simulink model "dataLoggerSimulink"  (R2023b)
settings: Solver=FixedStepDiscrete  StartTime=0.0  StopTime=10  FixedStep=50e-6  RelTol=1e-3
undefined symbols (not defined in the file or in its folder): A1, B1, fc, gamma, H1, H2, h3, J_dsmo, P, Te
libraries: embmathops x2
settings Model: Creator=salhajhass  LastModifiedBy=rdelpoux

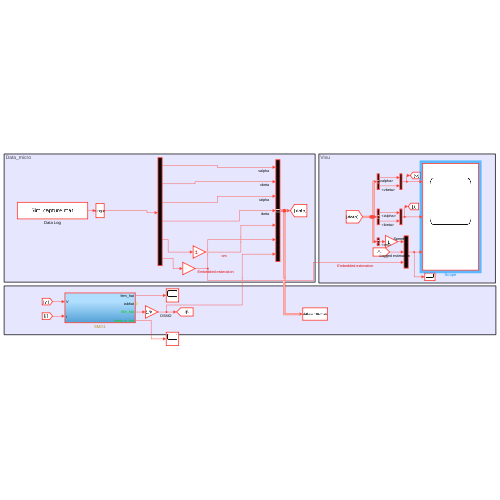
[thumbnail: Simulink's stored preview of the top-level diagram]
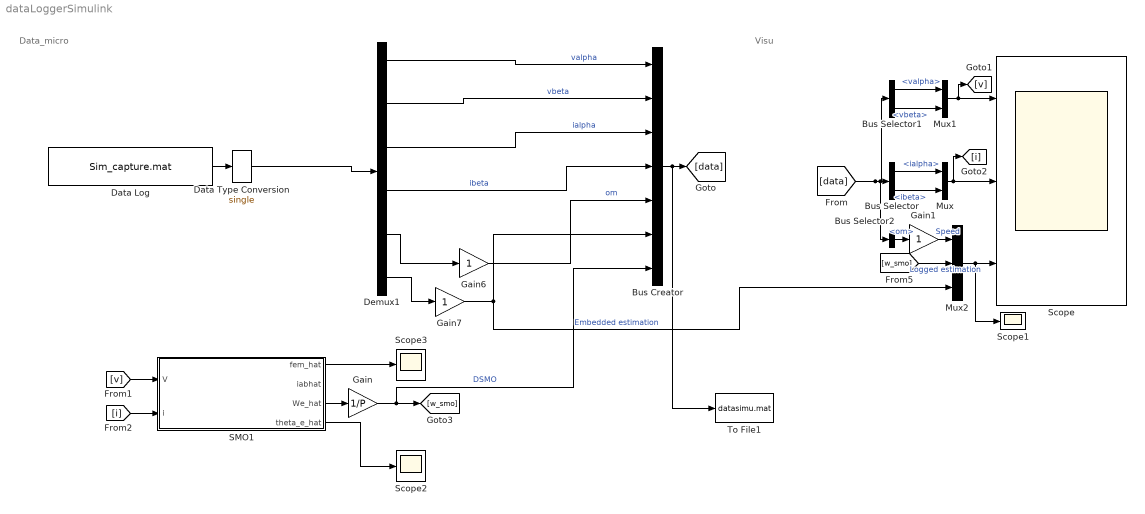
== system dataLoggerSimulink ==
  note: Visu
  note: Data_micro
  Bus Creator : BusCreator  Inputs=7
  Bus Selector : BusSelector  OutputSignals=ialpha,ibeta
  Bus Selector1 : BusSelector  OutputSignals=valpha,vbeta
  Bus Selector2 : BusSelector  OutputSignals=om
  Data Log : FromFile  FileName=Sim_capture.mat  SampleTime=50e-6
  Data Type Conversion : DataTypeConversion  OutDataTypeStr=single  SaturateOnIntegerOverflow=off  RndMeth=Floor
  Demux1 : Demux  Outputs=6
  Gain : Gain  Gain=1/P
  Gain1 : Gain
  Gain6 : Gain  OutDataTypeStr=single
  Gain7 : Gain  OutDataTypeStr=single
  Mux : Mux  Inputs=2
  Mux1 : Mux  Inputs=2
  Mux2 : Mux  Inputs=3
  SMO1 : Subsystem
  Scope : Scope  NumInputPorts=3
  Scope1 : Scope
  Scope2 : Scope
  Scope3 : Scope
  To File1 : ToFile  Filename=datasimu.mat  SaveFormat=Timeseries  SampleTime=5e-5
  wires:
  Data Log/1 -> Data Type Conversion/1
  Demux1/5 -> Gain6/1
  Bus Creator/1 -> To File1/1, [data]
  Bus Selector/1 -> Mux/1  "<ialpha>"
  Bus Selector/2 -> Mux/2  "<ibeta>"
  Mux/1 -> [i], Scope/2
  Mux1/1 -> [v], Scope/1
  Bus Selector1/2 -> Mux1/2  "<vbeta>"
  Bus Selector1/1 -> Mux1/1  "<valpha>"
  [data] -> Bus Selector1/1, Bus Selector2/1, Bus Selector/1
  Mux2/1 -> Scope1/1, Scope/3
  SMO1/3(We_hat) -> Gain/1
  Gain6/1 -> Bus Creator/5  "om"
  [v] -> SMO1/1(V)
  [i] -> SMO1/2(i)
  Gain/1 -> Bus Creator/7, [w_smo]  "DSMO"
  [w_smo] -> Mux2/2  "Logged estimation"
  Data Type Conversion/1 -> Demux1/1
  Demux1/3 -> Bus Creator/3  "ialpha"
  Demux1/4 -> Bus Creator/4  "ibeta"
  Demux1/2 -> Bus Creator/2  "vbeta"
  Demux1/1 -> Bus Creator/1  "valpha"
  Demux1/6 -> Gain7/1
  Gain7/1 -> Bus Creator/6, Mux2/3  "Embedded estimation"
  SMO1/1(fem_hat) -> Scope3/1
  Bus Selector2/1 -> Gain1/1  "<om>"
  Gain1/1 -> Mux2/1  "Speed"
  SMO1/4(theta_e_hat) -> Scope2/1

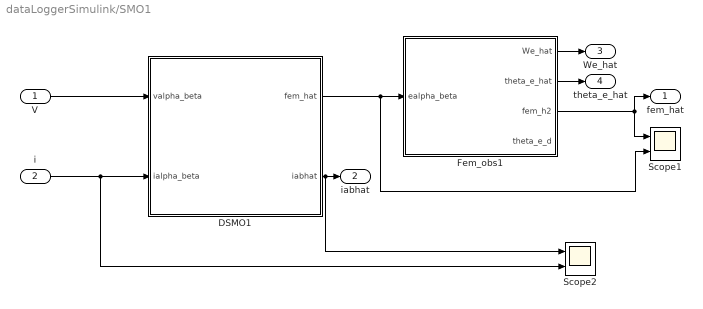
== system dataLoggerSimulink/SMO1 ==
  V : Inport
  i : Inport  Port=2
  DSMO1 : Subsystem
  Fem_obs1 : Subsystem
  Scope1 : Scope  NumInputPorts=2
  Scope2 : Scope  NumInputPorts=2
  fem_hat : Outport
  iabhat : Outport  Port=2
  We_hat : Outport  Port=3
  theta_e_hat : Outport  Port=4
  wires:
  Fem_obs1/3(fem_h2) -> fem_hat/1, Scope1/1
  Fem_obs1/2(theta_e_hat) -> theta_e_hat/1
  Fem_obs1/1(We_hat) -> We_hat/1
  i/1 -> Scope2/2, DSMO1/2(ialpha_beta)
  V/1 -> DSMO1/1(valpha_beta)
  DSMO1/2(iabhat) -> Scope2/1, iabhat/1
  DSMO1/1(fem_hat) -> Fem_obs1/1(ealpha_beta), Scope1/2

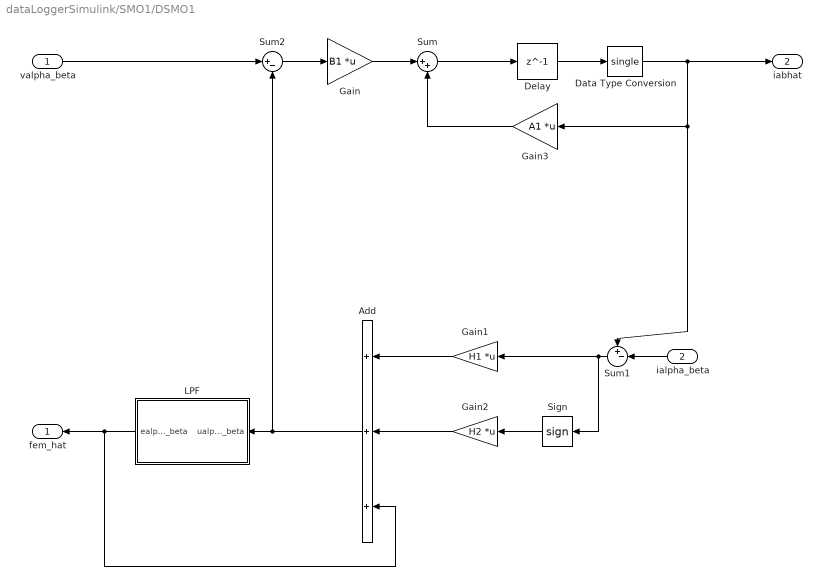
== system dataLoggerSimulink/SMO1/DSMO1 ==
  valpha_beta : Inport
  ialpha_beta : Inport  Port=2
  Add : Sum  Inputs=+++
  Data Type Conversion : DataTypeConversion  OutDataTypeStr=single  SaturateOnIntegerOverflow=off  RndMeth=Floor
  Delay : Delay  DelayLength=1  InitialCondition=0  SampleTime=Te
  Gain : Gain  Gain=B1  Multiplication=Matrix(K*u)
  Gain1 : Gain  Gain=H1  Multiplication=Matrix(K*u)
  Gain2 : Gain  Gain=H2  Multiplication=Matrix(K*u)
  Gain3 : Gain  Gain=A1  Multiplication=Matrix(K*u)
  LPF : Subsystem
  Sign : Signum
  Sum : Sum  Inputs=|++
  Sum1 : Sum  Inputs=+-|
  Sum2 : Sum  Inputs=|+-
  fem_hat : Outport
  iabhat : Outport  Port=2
  wires:
  Data Type Conversion/1 -> Gain3/1, Sum1/1, iabhat/1
  Delay/1 -> Data Type Conversion/1
  Add/1 -> Sum2/2, LPF/1(ualpha_beta)
  LPF/1(ealpha_beta) -> fem_hat/1, Add/3
  Gain2/1 -> Add/2
  Sign/1 -> Gain2/1
  Gain1/1 -> Add/1
  Sum1/1 -> Gain1/1, Sign/1
  valpha_beta/1 -> Sum2/1
  Sum2/1 -> Gain/1
  ialpha_beta/1 -> Sum1/2
  Gain3/1 -> Sum/2
  Gain/1 -> Sum/1
  Sum/1 -> Delay/1

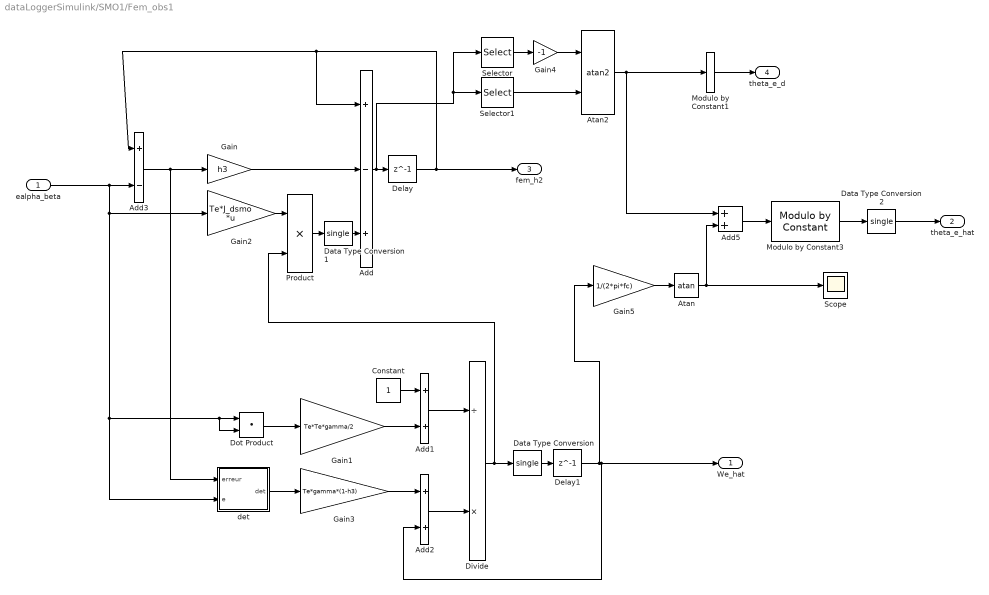
== system dataLoggerSimulink/SMO1/Fem_obs1 ==
  ealpha_beta : Inport
  Add : Sum  Inputs=+-+
  Add1 : Sum
  Add2 : Sum
  Add3 : Sum  Inputs=+-
  Add5 : Sum
  Atan : Trigonometry  Operator=atan
  Atan2 : Trigonometry  Operator=atan2  ApproximationMethod=Lookup  NumberOfDataPoints=32
  Constant : Constant
  Data Type Conversion : DataTypeConversion  OutDataTypeStr=single  SaturateOnIntegerOverflow=off  RndMeth=Floor
  Data Type Conversion1 : DataTypeConversion  OutDataTypeStr=single  SaturateOnIntegerOverflow=off  RndMeth=Floor
  Data Type Conversion2 : DataTypeConversion  OutDataTypeStr=single  SaturateOnIntegerOverflow=off  RndMeth=Floor
  Delay : Delay  DelayLength=1  SampleTime=Te
  Delay1 : Delay  DelayLength=1  SampleTime=Te
  Divide : Product  Inputs=/*
  Dot Product : DotProduct  OutDataTypeStr=Inherit: Inherit via internal rule
  Gain : Gain  Gain=h3
  Gain1 : Gain  Gain=Te*Te*gamma/2
  Gain2 : Gain  Gain=Te*J_dsmo  Multiplication=Matrix(K*u)
  Gain3 : Gain  Gain=Te*gamma*(1-h3)
  Gain4 : Gain  Gain=-1
  Gain5 : Gain  Gain=1/(2*pi*fc)
  Modulo by Constant1 : embmathops/Modulo by Constant  Denominator=2*pi  SimulateUsing=Code generation
      settings: LibrarySourceBlock=embeddedMathLib/Modulo by Constant
  Modulo by Constant3 : embmathops/Modulo by Constant  Denominator=2*pi  SimulateUsing=Code generation
      settings: LibrarySourceBlock=embeddedMathLib/Modulo by Constant
  Product : Product
  Scope : Scope
  Selector : Selector  InputPortWidth=2  IndexOptions=Index vector (dialog)  Indices=[1]  OutputSizes=1
  Selector1 : Selector  InputPortWidth=2  IndexOptions=Index vector (dialog)  Indices=2  OutputSizes=1
  det : Subsystem
  We_hat : Outport
  theta_e_hat : Outport  Port=2
  fem_h2 : Outport  Port=3
  theta_e_d : Outport  Port=4
  wires:
  Data Type Conversion2/1 -> theta_e_hat/1
  Data Type Conversion1/1 -> Add/3
  Product/1 -> Data Type Conversion1/1
  Divide/1 -> Data Type Conversion/1, Product/2
  Data Type Conversion/1 -> Delay1/1
  Modulo by Constant1/1 -> theta_e_d/1
  Delay1/1 -> Add2/2, We_hat/1, Gain5/1
  Modulo by Constant3/1 -> Data Type Conversion2/1
  Add5/1 -> Modulo by Constant3/1
  Gain5/1 -> Atan/1
  Constant/1 -> Add1/1
  Atan/1 -> Add5/2, Scope/1
  Atan2/1 -> Add5/1, Modulo by Constant1/1
  Selector1/1 -> Atan2/2
  Gain4/1 -> Atan2/1
  Selector/1 -> Gain4/1
  Gain/1 -> Add/2
  ealpha_beta/1 -> Add3/2, Gain2/1, det/2(e), Dot Product/1, Dot Product/2
  Gain3/1 -> Add2/1
  det/1(det) -> Gain3/1
  Add2/1 -> Divide/2
  Gain1/1 -> Add1/2
  Add1/1 -> Divide/1
  Dot Product/1 -> Gain1/1
  Delay/1 -> fem_h2/1, Add3/1, Add/1
  Add/1 -> Selector/1, Selector1/1, Delay/1
  Gain2/1 -> Product/1
  Add3/1 -> det/1(erreur), Gain/1

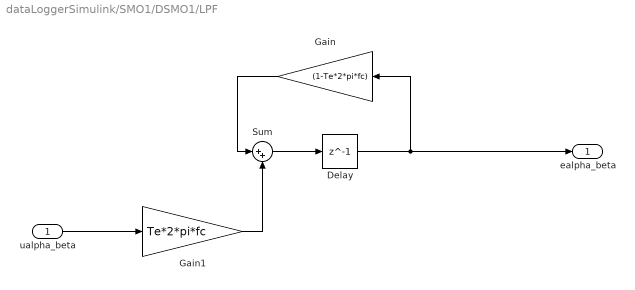
== system dataLoggerSimulink/SMO1/DSMO1/LPF ==
  ualpha_beta : Inport
  Delay : Delay  DelayLength=1  SampleTime=Te
  Gain : Gain  Gain=(1-Te*2*pi*fc)
  Gain1 : Gain  Gain=Te*2*pi*fc
  Sum : Sum  Inputs=|++
  ealpha_beta : Outport
  wires:
  ualpha_beta/1 -> Gain1/1
  Gain1/1 -> Sum/2
  Gain/1 -> Sum/1
  Delay/1 -> ealpha_beta/1, Gain/1
  Sum/1 -> Delay/1

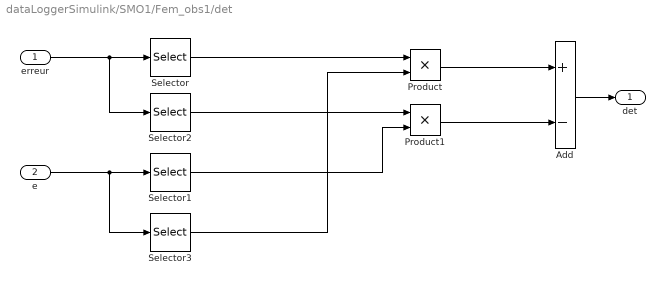
== system dataLoggerSimulink/SMO1/Fem_obs1/det ==
  erreur : Inport
  e : Inport  Port=2
  Add : Sum  Inputs=+-
  Product : Product
  Product1 : Product
  Selector : Selector  InputPortWidth=2  IndexOptions=Index vector (dialog)  Indices=[1]  OutputSizes=1
  Selector1 : Selector  InputPortWidth=2  IndexOptions=Index vector (dialog)  Indices=[1]  OutputSizes=1
  Selector2 : Selector  InputPortWidth=2  IndexOptions=Index vector (dialog)  Indices=[2]  OutputSizes=1
  Selector3 : Selector  InputPortWidth=2  IndexOptions=Index vector (dialog)  Indices=[2]  OutputSizes=1
  det : Outport
  wires:
  Add/1 -> det/1
  Product1/1 -> Add/2
  Selector1/1 -> Product1/2
  Selector2/1 -> Product1/1
  Product/1 -> Add/1
  Selector3/1 -> Product/2
  Selector/1 -> Product/1
  e/1 -> Selector1/1, Selector3/1
  erreur/1 -> Selector/1, Selector2/1
